simulink model "task3_lab2"  (R2020b)
settings: Solver=VariableStepAuto  StartTime=0.0  StopTime=0.3  RelTol=1e-3  EnableMultiTasking=on
settings Model: Creator=JackShen  LastModifiedBy=mluser
settings DataIOCC: LimitDataPoints=on  ReturnWorkspaceOutputs=off
settings OptimizationCC: LifeSpan=inf
settings DebuggingCC: AllowSymbolicDim=off  SFUnexpectedBacktrackingDiag=warning  SFNoUnconditionalDefaultTransitionDiag=warning  SFExecutionAtInitializationDiag=none  ArithmeticOperatorsInVariantConditions=warning
settings ModelReferenceCC: PropagateSignalLabelsOutOfModel=off
settings SFSimCC: SimUseLocalCustomCode=off  CustomCodeUndefinedFunction=UseInterfaceOnly
settings RTWCC: RTWUseLocalCustomCode=off
settings CodeAppCC: StateflowObjectComments=on
settings GRTTargetCC: TargetLangStandard=C89/C90 (ANSI)
settings ConfigComp: CovMetricSettings=dw  CovSaveCumulativeToWorkspaceVar=on  CovSaveSingleToWorkspaceVar=on  CovExternalEMLEnable=off

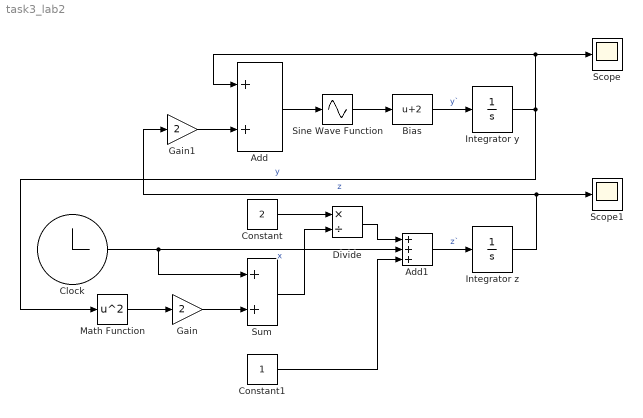
== system task3_lab2 ==
  Add : Sum
  Add1 : Sum  Inputs=+++
  Bias : Bias  Bias=2
  Clock : Clock
  Constant : Constant  Value=2
  Constant1 : Constant
  Divide : Product  Inputs=*/
  Gain : Gain  Gain=2
  Gain1 : Gain  Gain=2
  Integrator y : Integrator  InitialCondition=1
  Integrator z : Integrator  InitialCondition=0.05
  Math Function : Math  Operator=square  SignedPower=on  SaturateOnIntegerOverflow=on
  Scope : Scope
  Scope1 : Scope
  Sine Wave Function : Sin  TimeSource=Use external signal  Phase=pi/2  SampleTime=0
  Sum : Sum
  wires:
  Bias/1 -> Integrator y/1  "y`"
  Add1/1 -> Integrator z/1  "z`"
  Sine Wave Function/1 -> Bias/1
  Add/1 -> Sine Wave Function/1
  Gain1/1 -> Add/2
  Integrator z/1 -> Scope1/1, Gain1/1  "z"
  Constant/1 -> Divide/1
  Math Function/1 -> Gain/1
  Gain/1 -> Sum/2
  Sum/1 -> Divide/2
  Integrator y/1 -> Scope/1, Add/1, Math Function/1  "y"
  Constant1/1 -> Add1/3
  Clock/1 -> Sum/1, Add1/2  "x"
  Divide/1 -> Add1/1
